simulink model "power_simplealt"  (Simulink 6.0)
settings: Solver=ode23tb  SolverMode=SingleTasking  StartTime=0.0  StopTime=2  FixedStep=1e-3  RelTol=1e-3
libraries: powerlib x5, powerlib_extras x2
settings Model: Creator=patrice  LastModifiedBy=batserve  ExtModeTrigMode=oneshot  ExtModeArmWhenConnect=off  ExtModeAutoUpdateStatusClock=off
settings DataIOCC: InitialState=xinit  LimitDataPoints=off  SaveOutput=off  TimeSaveName=t  SignalLoggingName=sigsOut
settings OptimizationCC: BooleanDataType=off
settings DebuggingCC: SolverPrmCheckMsg=none  UnconnectedInputMsg=none  UnconnectedOutputMsg=none
settings HardwareCC: TargetUnknown=on
settings RTWCC: TemplateMakefile=grt_unix.tmf

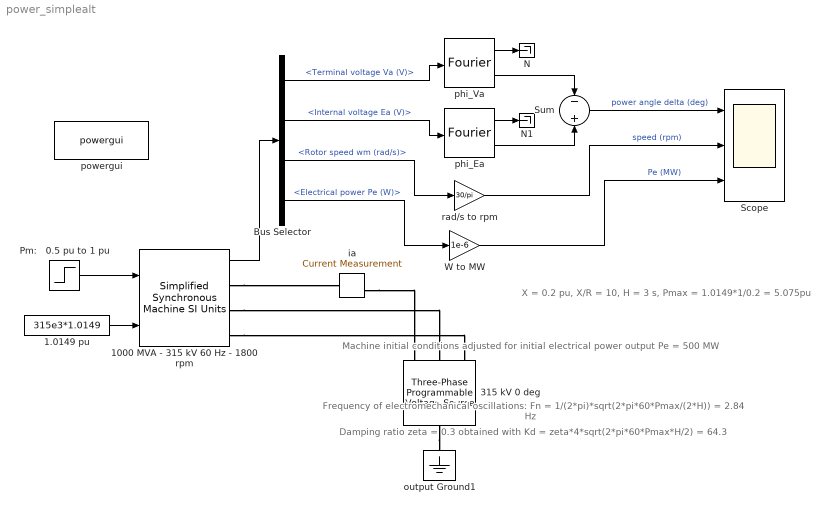
== system power_simplealt ==
  note: Machine  initial conditions adjusted
      | for initial  electrical power output Pe = 500 MW
  note: X = 0.2 pu, X/R = 10, H = 3 s, Pmax = 1.0149*1/0.2 = 5.075pu
  note: Frequency of electromechanical oscillations:
      | Fn = 1/(2*pi)*sqrt(2*pi*60*Pmax/(2*H)) = 2.84 Hz
  note: Damping ratio zeta = 0.3 obtained with
      | Kd = zeta*4*sqrt(2*pi*60*Pmax*H/2) = 64.3
  1.0149 pu : Constant  Value=315e3*1.0149
  1000 MVA - 315 kV 60 Hz - 1800 rpm : powerlib/Machines/Simplified Synchronous Machine SI Units  ConnectionType=3-wire Y  NominalParameters=[ 1000e6, 315e3, 60 ]  Mechanical="[168870,  64.3,  2]"  InternalRL=[ 99.225*0.02 ,99.225/(2*pi*60)*0.2 ]  InitialConditions=[0 5.65442 1296.03 1296.03 1296.03 0 -120 120]  Units=1  LoadFlowParameters=[1 500000000 0 0 0]
      settings: AttributesFormatString=\n
  315 kV 0 deg : powerlib/Electrical Sources/Three-Phase Programmable Voltage Source  Orientation=up  PositiveSequence="[315e3 0  60]"  VariationEntity=None  VariationType=Step  VariationStep=-0.5  VariationRate=10  VariationMagnitude=0.3  VariationFrequency=2  VariationTiming=[0.1 1.2]  VariationPhaseA=off  Amplitudes=[1 0.8 1.2 1.0]  TimeValues=[0 0.1 0.15 0.2]  HarmonicGeneration=off  HarmonicA=[3 0.2 -25 0]  HarmonicB="[2 0.15  35 2]"  Timing="[0.05  3]"
  Bus Selector : BusSelector  DialogController=Simulink.DDGSource_Bus  OutputSignals=Terminal voltage Va (V),Internal voltage Ea (V),Rotor speed wm (rad/s),Electrical power Pe (W)
  N : Terminator
  N1 : Terminator
  Pm:   0.5 pu to 1 pu : Step  Time=0.5  Before=505e6  After=1000e6  SampleTime=0
  Scope : Scope  NumInputPorts=3
      settings: YMin=5~1797~500  YMax=14~1806~1200  SaveName=delta  DataFormat=Structure
  Sum : Sum  Inputs=-+  SaturateOnIntegerOverflow=on  InputSameDT=on
  W to MW : Gain  Gain=1e-6  SaturateOnIntegerOverflow=on
  ia : powerlib/Measurements/Current Measurement  Tag=PoWeRsYsTeMmEaSuReMeNt  PhasorSimulation=off  OutputType=Magnitude  PSBequivalent=0
  output Ground1 : powerlib/Elements/Ground  Orientation=down  PhysicalDomain=powersysdomain  SubClassName=unknown  LeftPortType=p1  RightPortType=p1  LConnTagsString=a
  phi_Ea : powerlib_extras/Measurements/Fourier  f1=60  n=1
  phi_Va : powerlib_extras/Measurements/Fourier  f1=60  n=1
  powergui : powerlib/powergui  Priority=2  Frange=[0:2:500]  Ylog=off  Xlog=off  save=off  variable=ZData  ZoomFFT=on  StartTime=0.0  cycles=1  DisplayStyle=off  fundamental=60  FreqAxis=off  MaxFrequency=1000  frequencyindice=60  frequencyindicesteady=1  RmsSteady=1  display=off  Ts=0  methode=off  frequency=60  echomessages=off
  rad/s to rpm : Gain  Gain=30/pi  SaturateOnIntegerOverflow=on
  wires:
  rad/s to rpm/1 -> Scope/2  "speed (rpm)"
  W to MW/1 -> Scope/3  "Pe (MW)"
  phi_Va/2 -> Sum/1
  phi_Ea/2 -> Sum/2
  Sum/1 -> Scope/1  "power angle delta (deg)"
  phi_Va/1 -> N/1
  phi_Ea/1 -> N1/1
  Pm:   0.5 pu to 1 pu/1 -> 1000 MVA - 315 kV 60 Hz - 1800 rpm/1
  1.0149 pu/1 -> 1000 MVA - 315 kV 60 Hz - 1800 rpm/2
  1000 MVA - 315 kV 60 Hz - 1800 rpm/1 -> Bus Selector/1
  Bus Selector/1 -> phi_Va/1  "<Terminal voltage Va (V)>"
  Bus Selector/2 -> phi_Ea/1  "<Internal voltage Ea (V)>"
  Bus Selector/3 -> rad/s to rpm/1  "<Rotor speed wm (rad/s)>"
  Bus Selector/4 -> W to MW/1  "<Electrical power Pe (W)>"
  connections:
  1000 MVA - 315 kV 60 Hz - 1800 rpm/RConn1 -- ia/LConn1
  1000 MVA - 315 kV 60 Hz - 1800 rpm/RConn3 -- 315 kV 0 deg/RConn3
  ia/RConn1 -- 315 kV 0 deg/RConn1
  1000 MVA - 315 kV 60 Hz - 1800 rpm/RConn2 -- 315 kV 0 deg/RConn2
  315 kV 0 deg/LConn1 -- output Ground1/LConn1
